simulink model "FuzzyController"  (R2020b)
settings: Solver=VariableStepAuto  StartTime=0.0  StopTime=500  RelTol=1e-3
libraries: slctrlblks x1, fuzblock x1
settings Model: Creator=kumar  LastModifiedBy=kumar

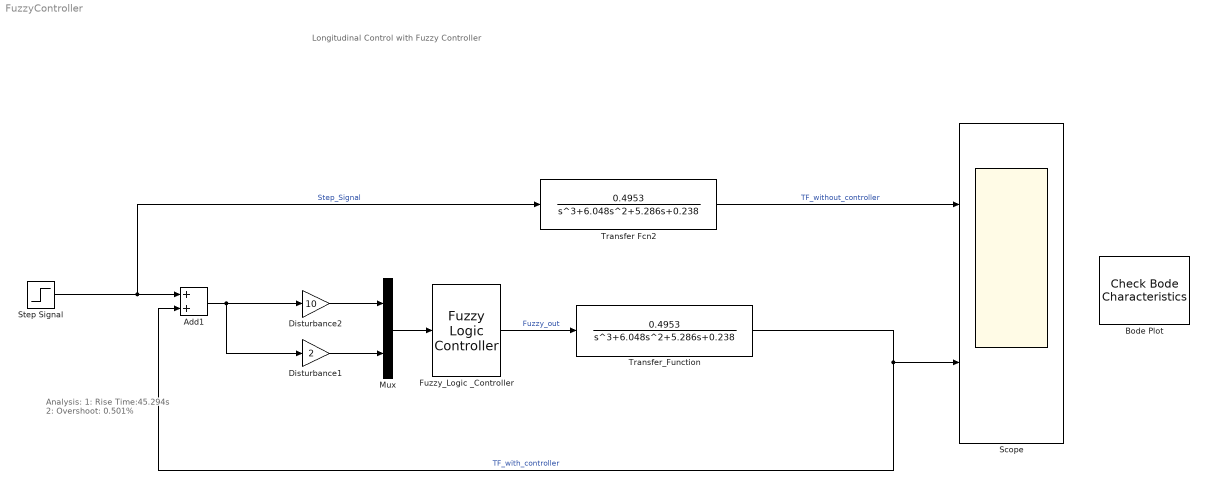
== system FuzzyController ==
  note: Analysis:
      | 1: Rise Time:45.294s
      | 2: Overshoot: 0.501%
  note: Longitudinal Control with Fuzzy Controller
  Add1 : Sum
  Bode Plot : slctrlblks/Model Verification/Check Bode  Characteristics  InstantiateOnLoad=on  SaveOperatingPoints=off  LinearizationIOs={'/Transfer_Function', 1, 'out', 'off', '';'/Step Signal', 1, 'in', 'off', ''}  LinearizeAt=SnapshotTimes  SnapshotTimes=[0]  TriggerType=rising  SampleTime=auto  RateConversionMethod=zoh  PreWarpFreq=10  UseExactDelayModel=off  UseFullBlockNameLabels=off  UseBusSignalLabels=off  enabled=on  stopWhenAssertionFail=off  export=off  ViewDlgPos=[1 41 1536 748.8]  OpenViewOnLoad=off  LaunchViewOnOpen=on  FrequencyUnits=rad/s  MagnitudeUnits=dB  PhaseUnits=deg  TimeUnits=seconds  EnableUpperBound=off  UpperBoundFrequencies=[]  UpperBoundMagnitudes=[]  EnableLowerBound=off  LowerBoundFrequencies=[]  LowerBoundMagnitudes=[]
  Disturbance1 : Gain  Gain=2
  Disturbance2 : Gain  Gain=10
  Fuzzy_Logic _Controller : fuzblock/Fuzzy Logic  Controller  FIS='tipper.fis'  OutputSampleNumber=101  DataType=double  FuzzifiedInputs=off  RuleFiringStrengths=off  RuleOutputs=off  AggregatedOutputs=off  SimulateUsing=Interpreted execution  OutOfRangeInputValueMessage=warning  NoRuleFiredMessage=warning  EmptyOutputFuzzySetMessage=warning
  Mux : Mux  Inputs=2
  Scope : Scope  NumInputPorts=2
  Step Signal : Step  SampleTime=0
  Transfer Fcn2 : TransferFcn  Numerator=0.4953  Denominator=[1 6.048 5.286 0.238]
  Transfer_Function : TransferFcn  Numerator=0.4953  Denominator=[1 6.048 5.286 0.238]
  wires:
  Step Signal/1 -> Transfer Fcn2/1, Add1/1  "Step_Signal"
  Disturbance2/1 -> Mux/1
  Disturbance1/1 -> Mux/2
  Mux/1 -> Fuzzy_Logic _Controller/1
  Fuzzy_Logic _Controller/1 -> Transfer_Function/1  "Fuzzy_out"
  Transfer_Function/1 -> Add1/2, Scope/2  "TF_with_controller"
  Transfer Fcn2/1 -> Scope/1  "TF_without_controller"
  Add1/1 -> Disturbance2/1, Disturbance1/1
